simulink model "ASKV9"  (R2024b)
settings: Solver=VariableStepAuto  StartTime=0.0  StopTime=0.05  RelTol=1e-3
libraries: spsFirstOrderFilterLib x31, simulink x6, simulink_extras x3, dspvision x1
settings Model: LastModifiedBy=fredy

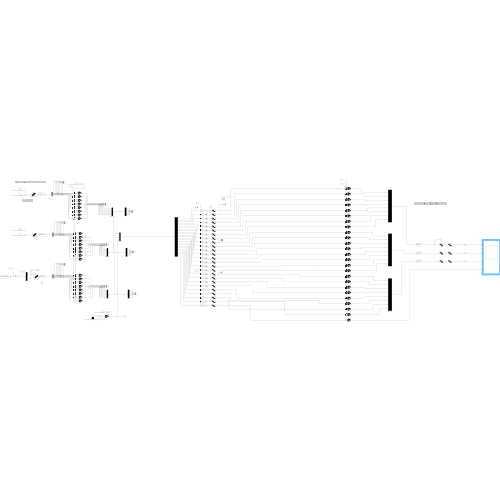
[thumbnail: Simulink's stored preview of the top-level diagram]
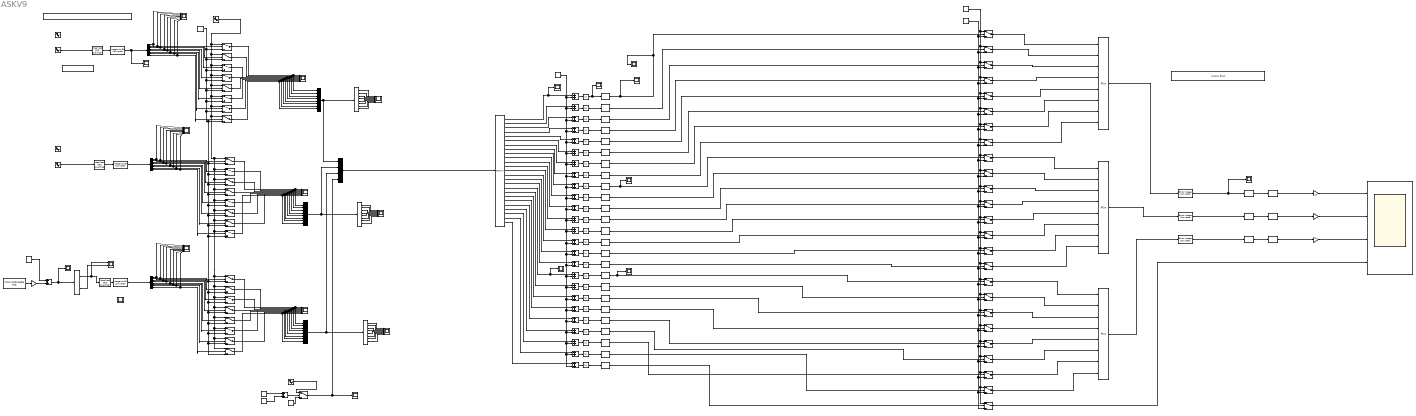
== system ASKV9 ==
  Abs{,1..24} (25 alike) : Abs  SaturateOnIntegerOverflow=off
  Add{,1..26} (27 alike) : Sum
  Bit to Integer Converter : simulink/Logic and Bit Operations/Bit to Integer Converter  nbits=8  bitOrder=MSB first  signedOutputValues=Unsigned  outDtype=Inherit via internal rule  outDtypeSigned=Inherit via internal rule
  Bit to Integer Converter1 : simulink/Logic and Bit Operations/Bit to Integer Converter  nbits=8  bitOrder=MSB first  signedOutputValues=Unsigned  outDtype=Inherit via internal rule  outDtypeSigned=Inherit via internal rule
  Bit to Integer Converter2 : simulink/Logic and Bit Operations/Bit to Integer Converter  nbits=8  bitOrder=MSB first  signedOutputValues=Unsigned  outDtype=Inherit via internal rule  outDtypeSigned=Inherit via internal rule
  Constant{,1..2,4} (4 alike) : Constant  Value=0.5
  Constant6 : Constant
  Constant7 : Constant  Value=-0.5
  Constant8 : Constant  Value=0
  Demux{,1..3,6..7} (6 alike) : Demux  Outputs=8
  Demux4 : Demux  Outputs=25
  Demux5 : Demux  Outputs=2
  Display : DisplayBlock  LabelPosition=Hide  Transparency=1  Layout=Fill available space
  Display1 : DisplayBlock  LabelPosition=Hide  Transparency=1
  Display2 : DisplayBlock  LabelPosition=Hide  Transparency=1
  First-Order Filter{,1..7,25..29,37} (14 alike) : spsFirstOrderFilterLib/First-Order Filter  FilterType=Lowpass  Tc=1.2e-6  Ts=0  Initialize=off  Vac_Init=[1, 0, 1000000]  Vdc_Init=0  PlotResponse=off  FreqRange="[0,  200,  1]"
  First-Order Filter{9..15} (7 alike) : spsFirstOrderFilterLib/First-Order Filter  FilterType=Lowpass  Tc=1.2e-6  Ts=0  Initialize=on  Vac_Init=[1, 0, 10000000]  Vdc_Init=0  PlotResponse=off  FreqRange="[0,  200,  1]"
  First-Order Filter{8,16..24} (10 alike) : spsFirstOrderFilterLib/First-Order Filter  FilterType=Lowpass  Tc=1.2e-6  Ts=0  Initialize=off  Vac_Init=[1, 0, 10000000]  Vdc_Init=0  PlotResponse=off  FreqRange="[0,  200,  1]"
  From Multimedia File1 : dspvision/From Multimedia File  inputFilename=D:\Datos Fredy\Programacion\Matlab\Modulacion ASK\audio.wav  readRange=[1 Inf]  loop=on  numPlays=inf  outputStreams=Audio only  videoDataType=single  audioDataType=single  inheritSampleTime=on  userDefinedSampleTime=1/30  noAudioOutput=off  isIntensityVideo=off  fourcc=RGB  colorVideoFormat=Separate color signals  outputEOF=off  dataOrg=Column-major  audioFrameSize=1  computeAudioFrameSize=off  outSamplingMode=Sample based
      settings: LibrarySourceBlock=audiosources/From Multimedia File
  Gain : Gain  Gain=500
  Gain1 : Gain  Gain=4e-3
  Gain2 : Gain  Gain=4e-3
  Gain3 : Gain  Gain=4e-3
  Idealized ADC quantizer : simulink_extras/Additional Discrete/Idealized ADC quantizer  NumberOfConverterBits=8  Vmin=0  Vmax=1  OutputDataType=double  OutputNegativeValues=off
  Idealized ADC quantizer1 : simulink_extras/Additional Discrete/Idealized ADC quantizer  NumberOfConverterBits=8  Vmin=0  Vmax=1  OutputDataType=double  OutputNegativeValues=off
  Idealized ADC quantizer2 : simulink_extras/Additional Discrete/Idealized ADC quantizer  NumberOfConverterBits=8  Vmin=0  Vmax=1  OutputDataType=double  OutputNegativeValues=off
  Integer to Bit Converter : simulink/Logic and Bit Operations/Integer to Bit Converter  nbits=8  signedInputValues=Unsigned  bitOrder=MSB first  outDtype=single
  Integer to Bit Converter1 : simulink/Logic and Bit Operations/Integer to Bit Converter  nbits=8  signedInputValues=Unsigned  bitOrder=MSB first  outDtype=Inherit via internal rule
  Integer to Bit Converter2 : simulink/Logic and Bit Operations/Integer to Bit Converter  nbits=8  signedInputValues=Unsigned  bitOrder=MSB first  outDtype=Inherit via internal rule
  Multiplexor (mux){,1,3..6} (6 alike) : Mux  Inputs=8
  Multiplexor (mux)2 : Mux
  Onda Cuadrada / Offset 0.5 / Amplitud 0.5 / Frecuencia 5K : SignalGenerator  WaveForm=square  Amplitude=0.5  Frequency=5000
  Onda Seno / Offset 0.5 / Amplitud 0.5 / Frecuencia 1 : Sin  Amplitude=0.5  Bias=0.5  Frequency=6.28321853071  SampleTime=0
  Onda Seno / Offset 0.5 / Amplitud 0.5 / Frecuencia 1.1 : Sin  Amplitude=0.5  Bias=0.5  Frequency=6.28321853071  SampleTime=0
  Onda Seno / Offset 0.5 / Amplitud 0.5 / Frecuencia 100K1 : Sin  Amplitude=0.5  Bias=0.5  Frequency=628318.5307  SampleTime=0
  Onda Seno / Offset 0.5 / Amplitud 0.5 / Frecuencia 10M : Sin  Amplitude=0.5  Bias=0.5  Frequency=62831853.07  SampleTime=0
  Onda Seno / Offset 0.5 / Amplitud 0.5 / Frecuencia 10k : Sin  Amplitude=0.5  Bias=0.5  Frequency=62831.853071  SampleTime=0
  Onda Seno / Offset 0.5 / Amplitud 0.5 / Frecuencia 1K : Sin  Amplitude=0.5  Bias=0.5  Frequency=6283.185307  SampleTime=0
  Scope{,7..8,12..15,17..20,22} (12 alike) : Scope
  Scope{1..6,10..11,21} (9 alike) : Scope  NumInputPorts=8
  Scope23 : Scope  NumInputPorts=4
  Scope9 : Scope  NumInputPorts=2
  Switch{,1..24} (25 alike) : Switch  Criteria=u2 > Threshold  Threshold=0.5  SaturateOnIntegerOverflow=off  InputSameDT=off
  Switch{25..49} (25 alike) : Switch  Criteria=u2 > Threshold  Threshold=.15  SaturateOnIntegerOverflow=off  InputSameDT=off
  wires:
  Constant/1 -> Add/1
  Onda Cuadrada / Offset 0.5 / Amplitud 0.5 / Frecuencia 5K/1 -> Add/2
  Add/1 -> Switch8/2
  Idealized ADC quantizer/1 -> Integer to Bit Converter/1
  Idealized ADC quantizer2/1 -> Integer to Bit Converter2/1
  Integer to Bit Converter2/1 -> Demux2/1
  Demux/1 -> Switch/2, Scope2/1
  Integer to Bit Converter/1 -> Scope15/1, Demux/1
  Demux/2 -> Switch1/2, Scope2/2
  Demux/3 -> Switch2/2, Scope2/3
  Demux/5 -> Switch4/2, Scope2/5
  Demux/4 -> Switch3/2, Scope2/4
  Demux/6 -> Switch5/2, Scope2/6
  Demux/7 -> Switch6/2, Scope2/7
  Demux/8 -> Switch7/2, Scope2/8
  Switch3/1 -> Multiplexor (mux)/4, Scope3/4
  Switch4/1 -> Multiplexor (mux)/5, Scope3/5
  Switch5/1 -> Multiplexor (mux)/6, Scope3/6
  Switch6/1 -> Multiplexor (mux)/7, Scope3/7
  Switch7/1 -> Multiplexor (mux)/8, Scope3/8
  Multiplexor (mux)/1 -> Multiplexor (mux)2/1, Demux1/1
  Demux1/1 -> Scope1/1
  Demux1/2 -> Scope1/2
  Demux1/3 -> Scope1/3
  Demux1/4 -> Scope1/4
  Demux1/5 -> Scope1/5
  Demux1/6 -> Scope1/6
  Demux1/7 -> Scope1/7
  Demux1/8 -> Scope1/8
  Constant2/1 -> Switch8/3
  Onda Seno / Offset 0.5 / Amplitud 0.5 / Frecuencia 100K1/1 -> Switch8/1
  Switch14/1 -> Multiplexor (mux)1/6, Scope6/6
  Switch15/1 -> Multiplexor (mux)1/7, Scope6/7
  Demux2/7 -> Switch15/2, Scope5/7
  Switch11/1 -> Multiplexor (mux)1/3, Scope6/3
  Demux2/3 -> Switch11/2, Scope5/3
  Demux2/6 -> Switch14/2, Scope5/6
  Demux2/5 -> Switch13/2, Scope5/5
  Demux2/8 -> Switch16/2, Scope5/8
  Demux2/4 -> Switch12/2, Scope5/4
  Demux2/1 -> Switch9/2, Scope5/1
  Switch9/1 -> Multiplexor (mux)1/1, Scope6/1
  Demux3/5 -> Scope4/5
  Demux3/8 -> Scope4/8
  Demux3/1 -> Scope4/1
  Switch10/1 -> Multiplexor (mux)1/2, Scope6/2
  Switch16/1 -> Multiplexor (mux)1/8, Scope6/8
  Switch13/1 -> Multiplexor (mux)1/5, Scope6/5
  Switch12/1 -> Multiplexor (mux)1/4, Scope6/4
  Demux3/6 -> Scope4/6
  Demux3/3 -> Scope4/3
  Demux3/2 -> Scope4/2
  Demux2/2 -> Switch10/2, Scope5/2
  Demux3/4 -> Scope4/4
  Demux3/7 -> Scope4/7
  Multiplexor (mux)2/1 -> Demux4/1
  Multiplexor (mux)1/1 -> Demux3/1, Multiplexor (mux)2/2
  Switch8/1 -> Multiplexor (mux)2/4, Scope8/1
  Constant4/1 -> Add1/1
  Switch19/1 -> Multiplexor (mux)3/4, Scope11/4
  Switch22/1 -> Multiplexor (mux)3/7, Scope11/7
  Switch20/1 -> Multiplexor (mux)3/5, Scope11/5
  Demux6/6 -> Switch21/2, Scope10/6
  Demux6/1 -> Switch24/2, Scope10/1
  Switch23/1 -> Multiplexor (mux)3/8, Scope11/8
  Demux6/5 -> Switch20/2, Scope10/5
  Onda Seno / Offset 0.5 / Amplitud 0.5 / Frecuencia 10M/1 -> Switch1/1, Switch2/1, Switch10/1, Switch11/1, Switch17/1, Switch18/1, Switch23/1, Switch22/1, Switch21/1, Switch20/1, Switch19/1, Switch24/1, Switch16/1, Switch15/1, Switch14/1, Switch13/1, Switch12/1, Switch9/1, Switch7/1, Switch6/1, Switch5/1, Switch4/1, Switch3/1, Switch/1
  Demux6/7 -> Switch22/2, Scope10/7
  Demux6/3 -> Switch18/2, Scope10/3
  Demux6/2 -> Switch17/2, Scope10/2
  Switch18/1 -> Multiplexor (mux)3/3, Scope11/3
  Demux6/8 -> Switch23/2, Scope10/8
  Switch17/1 -> Multiplexor (mux)3/2, Scope11/2
  Switch24/1 -> Multiplexor (mux)3/1, Scope11/1
  Constant1/1 -> Switch/3, Switch1/3, Switch2/3, Switch6/3, Switch10/3, Switch11/3, Switch15/3, Switch17/3, Switch18/3, Switch22/3, Switch23/3, Switch21/3, Switch20/3, Switch19/3, Switch24/3, Switch16/3, Switch14/3, Switch13/3, Switch12/3, Switch9/3, Switch7/3, Switch5/3, Switch4/3, Switch3/3
  Demux6/4 -> Switch19/2, Scope10/4
  Integer to Bit Converter1/1 -> Demux6/1
  Switch21/1 -> Multiplexor (mux)3/6, Scope11/6
  Multiplexor (mux)3/1 -> Demux7/1, Multiplexor (mux)2/3
  Constant6/1 -> Switch49/1, Switch48/1, Switch47/1, Switch46/1, Switch45/1, Switch44/1, Switch43/1, Switch42/1, Switch41/1, Switch40/1, Switch39/1, Switch38/1, Switch37/1, Switch36/1, Switch35/1, Switch34/1, Switch33/1, Switch32/1, Switch31/1, Switch30/1, Switch29/1, Switch28/1, Switch27/1, Switch26/1, Switch25/1
  Switch/1 -> Multiplexor (mux)/1, Scope3/1
  Switch1/1 -> Multiplexor (mux)/2, Scope3/2
  Switch2/1 -> Multiplexor (mux)/3, Scope3/3
  Add2/1 -> Abs/1
  Abs/1 -> Scope7/1, First-Order Filter/1
  Add3/1 -> Abs1/1
  Abs1/1 -> First-Order Filter1/1
  Add4/1 -> Abs2/1
  Abs2/1 -> First-Order Filter2/1
  Add5/1 -> Abs3/1
  Abs3/1 -> First-Order Filter3/1
  Add6/1 -> Abs4/1
  Abs4/1 -> First-Order Filter4/1
  Add7/1 -> Abs5/1
  Abs5/1 -> First-Order Filter5/1
  Add8/1 -> Abs6/1
  Abs6/1 -> First-Order Filter6/1
  Add9/1 -> Abs7/1
  Abs7/1 -> First-Order Filter7/1
  Add10/1 -> Abs8/1
  Abs8/1 -> First-Order Filter8/1
  Add11/1 -> Abs9/1
  Abs9/1 -> First-Order Filter9/1
  Add12/1 -> Abs10/1
  Abs10/1 -> First-Order Filter10/1
  Add13/1 -> Abs11/1
  Abs11/1 -> First-Order Filter11/1
  Add14/1 -> Abs12/1
  Abs12/1 -> First-Order Filter12/1
  Add15/1 -> Abs13/1
  Abs13/1 -> First-Order Filter13/1
  Add16/1 -> Abs14/1
  Abs14/1 -> First-Order Filter14/1
  Add17/1 -> Abs15/1
  Abs15/1 -> First-Order Filter15/1
  Add18/1 -> Abs16/1
  Abs16/1 -> First-Order Filter16/1
  Add19/1 -> Abs17/1
  Abs17/1 -> First-Order Filter17/1
  Add20/1 -> Abs18/1
  Abs18/1 -> First-Order Filter18/1
  Add21/1 -> Abs19/1
  Abs19/1 -> First-Order Filter19/1
  Add22/1 -> Abs20/1
  Abs20/1 -> First-Order Filter20/1
  Add23/1 -> Abs21/1
  Abs21/1 -> First-Order Filter21/1
  Add24/1 -> Abs22/1
  Abs22/1 -> First-Order Filter22/1
  Add25/1 -> Abs23/1
  Abs23/1 -> First-Order Filter23/1
  Add26/1 -> Abs24/1
  Abs24/1 -> First-Order Filter24/1
  Demux4/2 -> Add3/1
  Demux4/3 -> Add4/1
  Demux4/4 -> Add5/1
  Demux4/5 -> Add6/1
  Demux4/6 -> Add7/1
  Demux4/7 -> Add8/1
  Demux4/8 -> Add9/1
  Demux4/9 -> Add10/1
  Demux4/10 -> Add11/1
  Demux4/11 -> Add12/1
  Demux4/12 -> Add13/1
  Demux4/13 -> Add14/1
  Demux4/14 -> Add15/1
  Demux4/15 -> Add16/1
  Demux4/16 -> Add17/1
  Demux4/17 -> Scope20/1, Add18/1
  Demux4/18 -> Add19/1
  Demux4/19 -> Add20/1
  Demux4/20 -> Add21/1
  Demux4/21 -> Add22/1
  Demux4/22 -> Add23/1
  Demux4/23 -> Add24/1
  Demux4/24 -> Add25/1
  Demux4/25 -> Add26/1
  Demux4/1 -> Scope14/1, Add2/1
  Constant7/1 -> Add26/2, Add25/2, Add24/2, Add23/2, Add22/2, Add21/2, Add20/2, Add19/2, Add18/2, Add17/2, Add16/2, Add15/2, Add14/2, Add13/2, Add12/2, Add11/2, Add10/2, Add9/2, Add8/2, Add7/2, Add6/2, Add5/2, Add4/2, Add3/2, Add2/2
  Constant8/1 -> Switch49/3, Switch48/3, Switch47/3, Switch46/3, Switch45/3, Switch44/3, Switch43/3, Switch42/3, Switch41/3, Switch40/3, Switch39/3, Switch38/3, Switch37/3, Switch36/3, Switch35/3, Switch34/3, Switch33/3, Switch32/3, Switch31/3, Switch30/3, Switch29/3, Switch28/3, Switch27/3, Switch26/3, Switch25/3
  Switch25/1 -> Multiplexor (mux)4/1
  Switch26/1 -> Multiplexor (mux)4/2
  Switch27/1 -> Multiplexor (mux)4/3
  Switch28/1 -> Multiplexor (mux)4/4
  Switch29/1 -> Multiplexor (mux)4/5
  Switch30/1 -> Multiplexor (mux)4/6
  Switch31/1 -> Multiplexor (mux)4/7
  Switch32/1 -> Multiplexor (mux)4/8
  Switch33/1 -> Multiplexor (mux)5/1
  Switch34/1 -> Multiplexor (mux)5/2
  Switch35/1 -> Multiplexor (mux)5/3
  Switch36/1 -> Multiplexor (mux)5/4
  Switch37/1 -> Multiplexor (mux)5/5
  Switch38/1 -> Multiplexor (mux)5/6
  Switch39/1 -> Multiplexor (mux)5/7
  Switch40/1 -> Multiplexor (mux)5/8
  Switch41/1 -> Multiplexor (mux)6/1
  Switch42/1 -> Multiplexor (mux)6/2
  Switch43/1 -> Multiplexor (mux)6/3
  Switch44/1 -> Multiplexor (mux)6/4
  Switch45/1 -> Multiplexor (mux)6/5
  Switch46/1 -> Multiplexor (mux)6/6
  Switch47/1 -> Multiplexor (mux)6/7
  Switch48/1 -> Multiplexor (mux)6/8
  Multiplexor (mux)4/1 -> Bit to Integer Converter/1
  Multiplexor (mux)5/1 -> Bit to Integer Converter1/1
  Multiplexor (mux)6/1 -> Bit to Integer Converter2/1
  Switch49/1 -> Scope23/4
  Onda Seno / Offset 0.5 / Amplitud 0.5 / Frecuencia 1K/1 -> Idealized ADC quantizer2/1
  Onda Seno / Offset 0.5 / Amplitud 0.5 / Frecuencia 10k/1 -> Idealized ADC quantizer/1
  Demux7/5 -> Scope21/5
  Demux7/3 -> Scope21/3
  Demux7/1 -> Scope21/1
  Demux7/6 -> Scope21/6
  Demux7/4 -> Scope21/4
  Demux7/7 -> Scope21/7
  Demux7/2 -> Scope21/2
  Demux7/8 -> Scope21/8
  Add1/1 -> Scope22/1, Demux5/1
  From Multimedia File1/1 -> Gain/1
  Gain/1 -> Add1/2
  Demux5/1 -> Scope9/1, Idealized ADC quantizer1/1
  Demux5/2 -> Scope9/2
  Idealized ADC quantizer1/1 -> Integer to Bit Converter1/1
  First-Order Filter37/1 -> First-Order Filter29/1
  Bit to Integer Converter/1 -> First-Order Filter25/1, Scope13/1
  First-Order Filter26/1 -> First-Order Filter28/1
  Bit to Integer Converter2/1 -> First-Order Filter37/1
  Gain2/1 -> Scope23/2
  Gain1/1 -> Scope23/1
  Gain3/1 -> Scope23/3
  Bit to Integer Converter1/1 -> First-Order Filter26/1
  First-Order Filter/1 -> Scope/1, Scope17/1, Switch25/2
  First-Order Filter1/1 -> Switch26/2
  First-Order Filter11/1 -> Switch36/2
  First-Order Filter10/1 -> Switch35/2
  First-Order Filter17/1 -> Switch42/2
  First-Order Filter12/1 -> Switch37/2
  First-Order Filter14/1 -> Switch39/2
  First-Order Filter21/1 -> Switch46/2
  First-Order Filter19/1 -> Switch44/2
  First-Order Filter24/1 -> Switch49/2
  First-Order Filter18/1 -> Switch43/2
  First-Order Filter3/1 -> Switch28/2
  First-Order Filter16/1 -> Switch41/2, Scope19/1
  First-Order Filter2/1 -> Switch27/2
  First-Order Filter15/1 -> Switch40/2
  First-Order Filter13/1 -> Switch38/2
  First-Order Filter20/1 -> Switch45/2
  First-Order Filter9/1 -> Switch34/2
  First-Order Filter4/1 -> Switch29/2
  First-Order Filter7/1 -> Switch32/2
  First-Order Filter8/1 -> Switch33/2, Scope18/1
  First-Order Filter5/1 -> Switch30/2
  First-Order Filter6/1 -> Switch31/2
  First-Order Filter22/1 -> Switch47/2
  First-Order Filter23/1 -> Switch48/2
  First-Order Filter25/1 -> First-Order Filter27/1
  First-Order Filter27/1 -> Gain1/1
  First-Order Filter28/1 -> Gain2/1
  First-Order Filter29/1 -> Gain3/1
